simulink model "req20"  (R2019a)
settings: Solver=FixedStepAuto  StartTime=0.0  StopTime=100  RelTol=1e-3
libraries: simulink x3
settings Model: Creator=e40014285  LastModifiedBy=e40014285
settings ConfigComp: CovScope=ReferencedModels  CovHTMLOptions=-sRT=1 -sVT=0 -aTS=1 -bRG=1 -bTC=1 -hTR=0 -nFC=0 -nFD=1 -scm=1 -bcm=1 -xEv=0 -xEM=0  CovHtmlReporting=on  CovCumulativeReport=on  DVMaxProcessTime=6000  DVModelCoverageObjectives=EnhancedMCDC  DVTestSuiteOptimization=Auto  DVDetectOutOfBounds=on  DVReportPDFFormat=on  DVRebuildModelRepresentation=Always

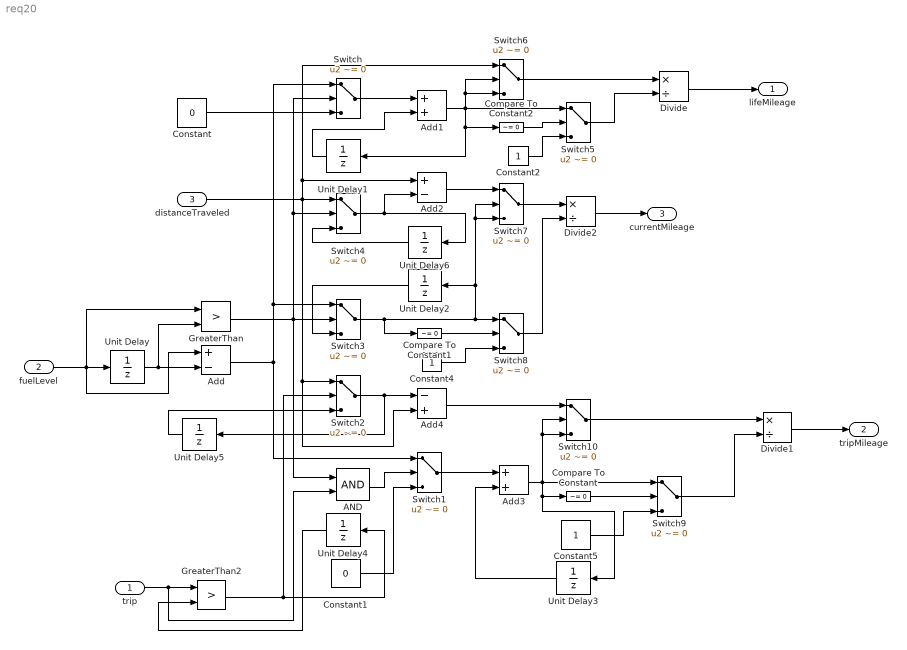
== system req20 ==
  trip : Inport
  fuelLevel : Inport  Port=2
  distanceTraveled : Inport  Port=3
  AND : Logic  AllPortsSameDT=off  OutDataTypeStr=boolean
  Add : Sum  Inputs=+-
  Add1 : Sum
  Add2 : Sum  Inputs=+-
  Add3 : Sum
  Add4 : Sum  Inputs=-+
  Compare To Constant : simulink/Logic and Bit Operations/Compare To Constant  relop=~=  const=0  OutDataTypeStr=boolean
  Compare To Constant1 : simulink/Logic and Bit Operations/Compare To Constant  relop=~=  const=0  OutDataTypeStr=boolean
  Compare To Constant2 : simulink/Logic and Bit Operations/Compare To Constant  relop=~=  const=0  OutDataTypeStr=boolean
  Constant : Constant  Value=0
  Constant1 : Constant  Value=0
  Constant2 : Constant
  Constant4 : Constant
  Constant5 : Constant
  Divide : Product  Inputs=*/
  Divide1 : Product  Inputs=*/
  Divide2 : Product  Inputs=*/
  GreaterThan : RelationalOperator  Operator=>  OutDataTypeStr=boolean  RndMeth=Simplest
  GreaterThan2 : RelationalOperator  Operator=>  OutDataTypeStr=boolean  RndMeth=Simplest
  Switch{,1..10} (11 alike) : Switch  Criteria=u2 ~= 0
  Unit Delay{,1..6} (7 alike) : UnitDelay  SampleTime=-1  HasFrameUpgradeWarning=on
  lifeMileage : Outport
  tripMileage : Outport  Port=2
  currentMileage : Outport  Port=3
  wires:
  Switch6/1 -> Divide/1
  Switch4/1 -> Add2/2, Unit Delay6/1
  Compare To Constant/1 -> Switch9/2
  Unit Delay6/1 -> Switch4/3
  Switch7/1 -> Divide2/1
  Constant5/1 -> Switch9/3
  Switch10/1 -> Divide1/1
  Compare To Constant2/1 -> Switch5/2
  Switch8/1 -> Divide2/2
  Compare To Constant1/1 -> Switch8/2
  Constant1/1 -> Switch1/3
  Unit Delay5/1 -> Switch2/3
  Divide1/1 -> tripMileage/1
  Switch9/1 -> Divide1/2
  GreaterThan/1 -> Switch4/2, Switch/2, AND/1, Switch3/2
  Unit Delay1/1 -> Add1/2
  Constant4/1 -> Switch8/3
  Unit Delay/1 -> Add/2, GreaterThan/2
  fuelLevel/1 -> Unit Delay/1, Add/1, GreaterThan/1
  Divide2/1 -> currentMileage/1
  Divide/1 -> lifeMileage/1
  Constant2/1 -> Switch5/3
  Switch5/1 -> Divide/2
  Switch/1 -> Add1/1
  Constant/1 -> Switch/3
  Unit Delay3/1 -> Add3/2
  Switch1/1 -> Add3/1
  Add4/1 -> Switch10/1
  Unit Delay2/1 -> Switch3/3
  Add3/1 -> Compare To Constant/1, Unit Delay3/1, Switch10/3, Switch10/2, Switch9/1
  GreaterThan2/1 -> Switch2/2, Unit Delay4/1
  AND/1 -> Switch1/2
  Unit Delay4/1 -> GreaterThan2/2
  Add2/1 -> Switch7/1
  Add1/1 -> Unit Delay1/1, Compare To Constant2/1, Switch6/3, Switch6/2, Switch5/1
  trip/1 -> GreaterThan2/1, AND/2
  distanceTraveled/1 -> Add4/2, Switch2/1, Add2/1, Switch6/1, Switch4/1
  Switch2/1 -> Add4/1, Unit Delay5/1
  Add/1 -> Switch3/1, Switch/1, Switch1/1
  Switch3/1 -> Switch7/3, Switch7/2, Unit Delay2/1, Switch8/1, Compare To Constant1/1
